simulink model "LgrstClsFlow"  (R2018b)
settings: Solver=FixedStepDiscrete  StartTime=0.0  StopTime=10.0  FixedStep=0.01  RelTol=1e-3
undefined symbols (not defined in the file or in its folder): KeSMSuSecRwStFtrstUpwdDnwdPosDelta_Val
settings Model: ModifiedHistory=v2.0.1腿托只发送目标位置  Creator=sn2xws  LastModifiedBy=sn55gm
settings DataIOCC: SaveFormat=StructureWithTime
settings OptimizationCC: DefaultParameterBehavior=Inlined  EnhancedBackFolding=on  PassReuseOutputArgsAs=Individual arguments  ZeroExternalMemoryAtStartup=off  ZeroInternalMemoryAtStartup=off  OptimizeBlockOrder=speed  DifferentSizesBufferReuse=on  OptimizationCustomize=off
settings DebuggingCC: ParameterTunabilityLossMsg=error
settings HardwareCC: ProdLongLongMode=on
settings SFSimCC: MATLABDynamicMemAlloc=off
settings RTWCC: SystemTargetFile=autosar.tlc  GenCodeOnly=on  TemplateMakefile=ert_default_tmf  Description=AUTOSAR  GenerateReport=on  IncludeHyperlinkInReport=on  LaunchReport=on  GenerateTraceInfo=on  GenerateTraceReport=on  GenerateTraceReportSl=on  GenerateTraceReportSf=on  GenerateTraceReportEml=on  GenerateCodeMetricsReport=on
settings CodeAppCC: ForceParamTrailComments=on  IgnoreCustomStorageClasses=off  OperatorAnnotations=on  SimulinkDataObjDesc=on  SFDataObjDesc=on  InsertBlockDesc=on
settings STFCustomTargetCC: TargetLangStandard=C99 (ISO)  MultiwordLength=256  ParMdlRefBuildCompliant=on  CompOptLevelCompliant=on  IncludeMdlTerminateFcn=off  CombineOutputUpdateFcns=on  SuppressErrorStatus=on  ERTCustomFileBanners=on  SupportNonFinite=off  SupportComplex=off  SupportContinuousTime=off  SupportNonInlinedSFcns=off  RemoveResetFunc=on  MATLABClassNameForMDSCustomization=Simulink.SoftwareTarget.ERTCustomization  AutosarCompliant=on  UseToolchainInfoCompliant=on  LookupTableObjectStructAxisOrder=2,1,3,4,...  LUTObjectStructOrderEvenSpacing=Size,Table,Breakpoints  SystemTargetFile=autosar.tlc
settings ERTTargetCC: TargetLangStandard=C99 (ISO)  ConcurrentExecutionCompliant=off  IncludeMdlTerminateFcn=off  SuppressErrorStatus=on  SupportNonFinite=off  SupportComplex=off  ModelStepFunctionPrototypeControlCompliant=off  CPPClassGenCompliant=off  AutosarCompliant=on  LookupTableObjectStructAxisOrder=2,1,3,4,...  LUTObjectStructOrderEvenSpacing=Size,Table,Breakpoints  InlinedParameterPlacement=NonHierarchical  ERTCustomFileTemplate=example_file_process.tlc  ERTFilePackagingFormat=Compact

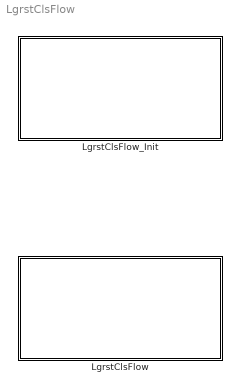
== system LgrstClsFlow ==
  LgrstClsFlow : Subsystem
  LgrstClsFlow_Init : Subsystem

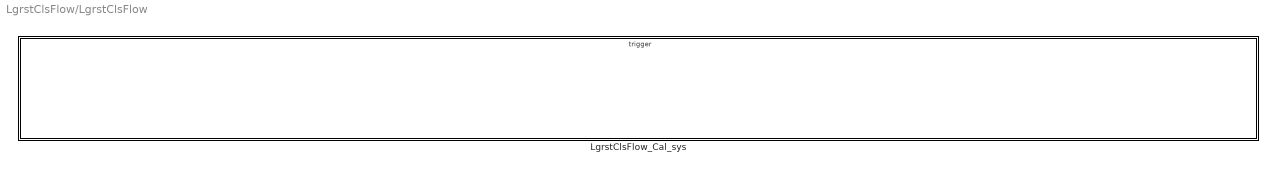
== system LgrstClsFlow/LgrstClsFlow ==
  LgrstClsFlow_Cal_sys : Subsystem

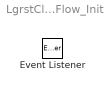
== system LgrstClsFlow/LgrstClsFlow_Init ==
  Event Listener : EventListener  EventName=reset

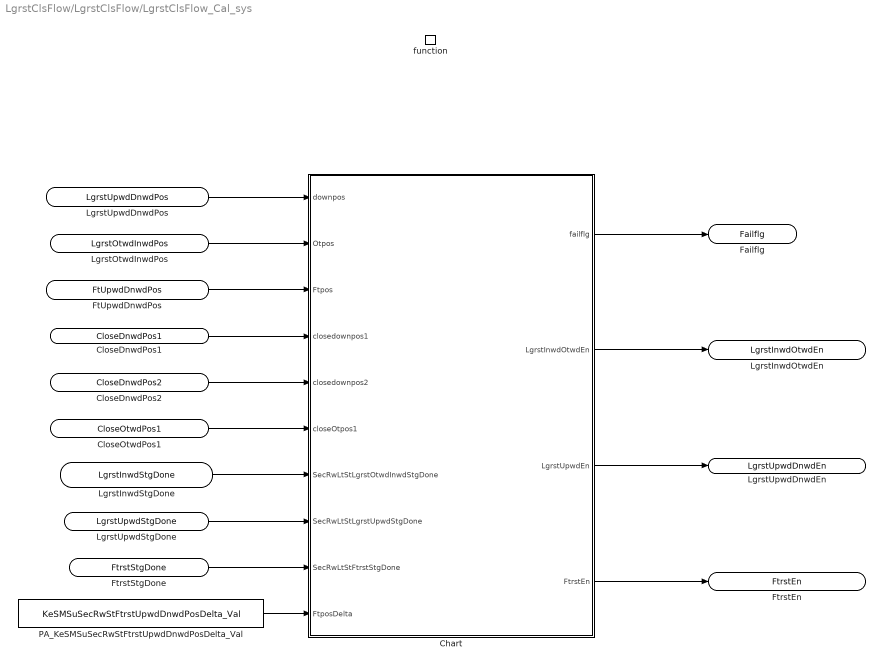
== system LgrstClsFlow/LgrstClsFlow/LgrstClsFlow_Cal_sys ==
  function : TriggerPort  TriggerType=function-call  IsSimulinkFunction=on  FunctionName=LgrstClsFlow_Cal  VariantControl=(inherit)
  Chart : Stateflow chart  TreatAsAtomicUnit=on
  PA_KeSMSuSecRwStFtrstUpwdDnwdPosDelta_Val : Constant  Value=KeSMSuSecRwStFtrstUpwdDnwdPosDelta_Val
  LgrstUpwdDnwdPos : ArgIn  OutDataTypeStr=uint16  ArgumentName=LgrstUpwdDnwdPos
  LgrstOtwdInwdPos : ArgIn  Port=2  OutDataTypeStr=uint16  ArgumentName=LgrstOtwdInwdPos
  FtUpwdDnwdPos : ArgIn  Port=3  OutDataTypeStr=uint16  ArgumentName=FtUpwdDnwdPos
  CloseDnwdPos1 : ArgIn  Port=4  OutDataTypeStr=uint16  ArgumentName=CloseDnwdPos1
  CloseDnwdPos2 : ArgIn  Port=5  OutDataTypeStr=uint16  ArgumentName=CloseDnwdPos2
  CloseOtwdPos1 : ArgIn  Port=6  OutDataTypeStr=uint16  ArgumentName=CloseOtwdPos1
  LgrstInwdStgDone : ArgIn  Port=7  OutDataTypeStr=boolean  ArgumentName=LgrstInwdStgDone
  LgrstUpwdStgDone : ArgIn  Port=8  OutDataTypeStr=boolean  ArgumentName=LgrstUpwdStgDone
  FtrstStgDone : ArgIn  Port=9  OutDataTypeStr=boolean  ArgumentName=FtrstStgDone
  Failflg : ArgOut  OutDataTypeStr=boolean  ArgumentName=Failflg
  LgrstInwdOtwdEn : ArgOut  Port=2  OutDataTypeStr=boolean  ArgumentName=LgrstInwdOtwdEn
  LgrstUpwdDnwdEn : ArgOut  Port=3  OutDataTypeStr=boolean  ArgumentName=LgrstUpwdDnwdEn
  FtrstEn : ArgOut  Port=4  OutDataTypeStr=boolean  ArgumentName=FtrstEn
  wires:
  PA_KeSMSuSecRwStFtrstUpwdDnwdPosDelta_Val/1 -> Chart/10(FtposDelta)
  Chart/1(failflg) -> Failflg/1
  LgrstUpwdDnwdPos/1 -> Chart/1(downpos)
  LgrstOtwdInwdPos/1 -> Chart/2(Otpos)
  FtUpwdDnwdPos/1 -> Chart/3(Ftpos)
  CloseDnwdPos1/1 -> Chart/4(closedownpos1)
  LgrstInwdStgDone/1 -> Chart/7(SecRwLtStLgrstOtwdInwdStgDone)
  CloseDnwdPos2/1 -> Chart/5(closedownpos2)
  CloseOtwdPos1/1 -> Chart/6(closeOtpos1)
  LgrstUpwdStgDone/1 -> Chart/8(SecRwLtStLgrstUpwdStgDone)
  FtrstStgDone/1 -> Chart/9(SecRwLtStFtrstStgDone)
  Chart/2(LgrstInwdOtwdEn) -> LgrstInwdOtwdEn/1
  Chart/4(FtrstEn) -> FtrstEn/1
  Chart/3(LgrstUpwdEn) -> LgrstUpwdDnwdEn/1

== stateflow chart LgrstClsFlow/LgrstClsFlow_Cal_sys/Chart ==
  (default) -> (junction 105) : {
      | failflg=0;
      | LgrstInwdOtwdEn=0;
      | LgrstUpwdEn=0;
      | FtrstEn=0;
      | }
  (junction 105) -> (junction 107) [order 1] : [SecRwLtStLgrstOtwdInwdStgDone]
  (junction 105) -> (junction 82) [order 2] : {
      | LgrstInwdOtwdEn=1;
      | }
  (junction 107) -> (junction 109)
  (junction 109) -> (junction 82)
  (junction 82) -> (junction 87)
  (junction 87) -> (junction 94) [order 1] : [SecRwLtStLgrstUpwdStgDone]
  (junction 87) -> (junction 91) [order 2] : {
      | LgrstUpwdEn=1;
      | }
  (junction 94) -> (junction 96)
  (junction 96) -> (junction 91)
  (junction 91) -> (junction 182)
  data: downpos input uint16; Otpos input uint16; Ftpos input uint16; closedownpos1 input uint16; closedownpos2 input uint16; closeOtpos1 input uint16; SecRwLtStLgrstOtwdInwdStgDone input boolean; SecRwLtStLgrstUpwdStgDone input boolean; SecRwLtStFtrstStgDone input boolean; FtposDelta input uint16; failflg output boolean; LgrstInwdOtwdEn output boolean; LgrstUpwdEn output boolean; FtrstEn output boolean
